simulink model "integrator_ext_reset_matrix_test_tmp"  (Simulink 8.3)
settings: Solver=ode45  StartTime=0.0  StopTime=10.0  RelTol=1e-3
undefined symbols (not defined in the file): DiscIntNeverNeededParam
settings Model: Creator=arnaud  LastModifiedBy=hbourbou
settings DataIOCC: SaveFormat=Structure
settings OptimizationCC: ExpressionDepthLimit=2147483647
settings DebuggingCC: FcnCallInpInsideContextMsg=EnableAllAsWarning  FrameProcessingCompatibilityMsg=error

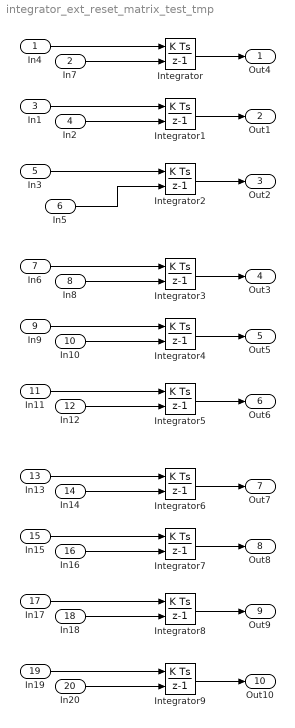
== system integrator_ext_reset_matrix_test_tmp ==
  In4 : Inport  OutDataTypeStr=double  PortDimensions=[2 2]
  In7 : Inport  Port=2  OutDataTypeStr=boolean
  In1 : Inport  Port=3  OutDataTypeStr=double
  In2 : Inport  Port=4  OutDataTypeStr=double  PortDimensions=[2 2]
  In3 : Inport  Port=5  OutDataTypeStr=int8  PortDimensions=[2 2]
  In5 : Inport  Port=6  OutDataTypeStr=int8  PortDimensions=[2 2]
  In6 : Inport  Port=7  OutDataTypeStr=double  PortDimensions=[2 2]
  In8 : Inport  Port=8  OutDataTypeStr=boolean
  In9 : Inport  Port=9  OutDataTypeStr=int32
  In10 : Inport  Port=10  OutDataTypeStr=int32  PortDimensions=[2 2]
  In11 : Inport  Port=11  OutDataTypeStr=double  PortDimensions=[2 2]
  In12 : Inport  Port=12  OutDataTypeStr=boolean  PortDimensions=[2 2]
  In13 : Inport  Port=13  OutDataTypeStr=double  PortDimensions=[2 2]
  In14 : Inport  Port=14  OutDataTypeStr=double
  In15 : Inport  Port=15  OutDataTypeStr=double
  In16 : Inport  Port=16  OutDataTypeStr=boolean  PortDimensions=[2 2]
  In17 : Inport  Port=17  OutDataTypeStr=double  PortDimensions=[2 2]
  In18 : Inport  Port=18  OutDataTypeStr=boolean  PortDimensions=[2 2]
  In19 : Inport  Port=19  OutDataTypeStr=double  PortDimensions=1
  In20 : Inport  Port=20  OutDataTypeStr=boolean
  Integrator : DiscreteIntegrator  ExternalReset=rising  SampleTime=1.0  ICPrevOutput=DiscIntNeverNeededParam  ICPrevScaledInput=DiscIntNeverNeededParam  mask(DiscretizedDiscreteIntegrator){}
      mask init:
      | %zoh
  Integrator1 : DiscreteIntegrator  ExternalReset=rising  SampleTime=1.0  ICPrevOutput=DiscIntNeverNeededParam  ICPrevScaledInput=DiscIntNeverNeededParam  mask(DiscretizedDiscreteIntegrator){}
      mask init:
      | %zoh
  Integrator2 : DiscreteIntegrator  ExternalReset=rising  SampleTime=1.0  ICPrevOutput=DiscIntNeverNeededParam  ICPrevScaledInput=DiscIntNeverNeededParam  mask(DiscretizedDiscreteIntegrator){}
      mask init:
      | %zoh
  Integrator3 : DiscreteIntegrator  ExternalReset=rising  InitialCondition=[25 54; .7 58]  SampleTime=1.0  ICPrevOutput=DiscIntNeverNeededParam  ICPrevScaledInput=DiscIntNeverNeededParam  mask(DiscretizedDiscreteIntegrator){}
      mask init:
      | %zoh
  Integrator4 : DiscreteIntegrator  ExternalReset=rising  InitialCondition=[25 54; .7 58]  SampleTime=1.0  ICPrevOutput=DiscIntNeverNeededParam  ICPrevScaledInput=DiscIntNeverNeededParam  mask(DiscretizedDiscreteIntegrator){}
      mask init:
      | %zoh
  Integrator5 : DiscreteIntegrator  ExternalReset=rising  InitialCondition=[25 54; .7 58]  SampleTime=1.0  ICPrevOutput=DiscIntNeverNeededParam  ICPrevScaledInput=DiscIntNeverNeededParam  mask(DiscretizedDiscreteIntegrator){}
      mask init:
      | %zoh
  Integrator6 : DiscreteIntegrator  gainval=[1 2; 3 4]  ExternalReset=rising  InitialCondition=[25 54; .7 58]  SampleTime=1.0  ICPrevOutput=DiscIntNeverNeededParam  ICPrevScaledInput=DiscIntNeverNeededParam  mask(DiscretizedDiscreteIntegrator){}
      mask init:
      | %zoh
  Integrator7 : DiscreteIntegrator  gainval=[1 2; 3 4]  ExternalReset=rising  InitialCondition=[25 54; .7 58]  SampleTime=1.0  ICPrevOutput=DiscIntNeverNeededParam  ICPrevScaledInput=DiscIntNeverNeededParam  mask(DiscretizedDiscreteIntegrator){}
      mask init:
      | %zoh
  Integrator8 : DiscreteIntegrator  gainval=[1 2; 3 4]  ExternalReset=rising  InitialCondition=[25 54; .7 58]  SampleTime=1.0  ICPrevOutput=DiscIntNeverNeededParam  ICPrevScaledInput=DiscIntNeverNeededParam  mask(DiscretizedDiscreteIntegrator){}
      mask init:
      | %zoh
  Integrator9 : DiscreteIntegrator  gainval=[1 2; 3 4]  ExternalReset=rising  InitialCondition=[25 54; .7 58]  SampleTime=1.0  ICPrevOutput=DiscIntNeverNeededParam  ICPrevScaledInput=DiscIntNeverNeededParam  mask(DiscretizedDiscreteIntegrator){}
      mask init:
      | %zoh
  Out4 : Outport
  Out1 : Outport  Port=2
  Out2 : Outport  Port=3
  Out3 : Outport  Port=4
  Out5 : Outport  Port=5
  Out6 : Outport  Port=6
  Out7 : Outport  Port=7
  Out8 : Outport  Port=8
  Out9 : Outport  Port=9
  Out10 : Outport  Port=10
  wires:
  In4/1 -> Integrator/1
  Integrator/1 -> Out4/1
  In7/1 -> Integrator/2
  In1/1 -> Integrator1/1
  Integrator1/1 -> Out1/1
  In2/1 -> Integrator1/2
  In3/1 -> Integrator2/1
  Integrator2/1 -> Out2/1
  In5/1 -> Integrator2/2
  In6/1 -> Integrator3/1
  Integrator3/1 -> Out3/1
  In8/1 -> Integrator3/2
  In9/1 -> Integrator4/1
  Integrator4/1 -> Out5/1
  In10/1 -> Integrator4/2
  In11/1 -> Integrator5/1
  Integrator5/1 -> Out6/1
  In12/1 -> Integrator5/2
  In13/1 -> Integrator6/1
  Integrator6/1 -> Out7/1
  In14/1 -> Integrator6/2
  In15/1 -> Integrator7/1
  Integrator7/1 -> Out8/1
  In16/1 -> Integrator7/2
  In17/1 -> Integrator8/1
  Integrator8/1 -> Out9/1
  In18/1 -> Integrator8/2
  In19/1 -> Integrator9/1
  Integrator9/1 -> Out10/1
  In20/1 -> Integrator9/2
